simulink model "MSDRPrimaryLoop_LoadFollow"  (R2021b)
settings: Solver=VariableStepAuto  StartTime=0.0  StopTime=604900  MaxStep=1  MinStep=0.01  RelTol=1e-3
undefined symbols (not defined in the file): a_f, A_free_PHX, a_g, A_h_PHX, beta, beta_t, bubbleGeneratorArea, bubbleGeneratorDh, bubbleGeneratorElevation, bubbleGeneratorLength, bubbleGeneratorVolume, bubbleSaturationLevel, bubbleSeparatorArea, bubbleSeparatorDiameter, bubbleSeparatorDo, bubbleSeparatorLength, bubbleSeparatorSlope, bypassRatio, C0, coreFlowArea, coreFuelVolume, coreLowerPlenumArea, coreLowerPlenumHydraulicDiameter, coreLowerPlenumLength, coreLowerPlenumVolume, coreUpperPlenumArea, coreUpperPlenumHydraulicDiameter, coreUpperPlenumLength, coreUpperPlenumVolume, coreVolume, cpGraphite, dissolusionRatio, dMin, dScale, dsmConst, DXeG, Fiss_factor, fuelChannelHydrualicDiameter, fuelChannelLength, fuelDepositRatio, fuelFraction, fuelGraphiteArea, fuelGraphiteHeatTransferCoefficient, gamma0, gamma1, gamma2, generatorDsm, graphiteKDiff, graphiteUnitCellThickness, initialIodineConcentration, InitialXeMolarConcentration, InjectionRatio, injectionRatio, iodineDecayConstant, IodineDecayConstant, iodineYield, kGraphite, kScale, Lam, lam ... (+60)
libraries: fl_lib x268, nesl_utility x106, SimscapeFluids_lib x20, slpidlib x1
(part 4 of 12)

== system MSDRPrimaryLoop_LoadFollow/pipeReactorToPump/PLossFunc ==
  Constant : Constant  Value=Elevation*9.82
  PS-Simulink Converter : nesl_utility/PS-Simulink Converter  PhysicalDomain=network_engine_domain  SubClassName=ps_output  LeftPortType=input  RightPortType=output  PseudoPeriodic=off  Frequencies=[]  Unit=inherit  AffineConversion=off
      settings: SourceProductBaseCode=PW,SS
  PS-Simulink Converter1 : nesl_utility/PS-Simulink Converter  PhysicalDomain=network_engine_domain  SubClassName=ps_output  LeftPortType=input  RightPortType=output  PseudoPeriodic=off  Frequencies=[]  Unit=inherit  AffineConversion=off
      settings: SourceProductBaseCode=PW,SS
  Pressure & Temperature Sensor (TL) : fl_lib/Thermal Liquid/Sensors/Pressure & Temperature Sensor (TL)
      settings: SourceProductBaseCode=SS  InternalSimscapePortConfiguration="{\"Bottom\":[],\"Left\":[{\"id\":\"A\",\"label\":\"A\",\"type\":\"foundation.thermal_liquid.thermal_liquid\"}],\"Right\":[{\"id\":\"B\",\"label\":\"B\",\"type\":\"foundation.thermal_liquid.thermal_liquid\"},{\"id\":\"P\",\"label\":\"P\",\"type\":\"output\"},{\"id\":\"T\",\"label\":\"T\",\"type\":\"output\"}],\"Top\":[]}"
  Product : Product
  Subtract : Sum  Inputs=+-
  Thermodynamic Properties Sensor (TL) : fl_lib/Thermal Liquid/Sensors/Thermodynamic Properties Sensor (TL)
      settings: SourceProductBaseCode=SS  InternalSimscapePortConfiguration="{\"Bottom\":[],\"Left\":[{\"id\":\"A\",\"label\":\"A\",\"type\":\"foundation.thermal_liquid.thermal_liquid\"}],\"Right\":[{\"id\":\"U\",\"label\":\"u\",\"type\":\"output\"},{\"id\":\"RHO\",\"label\":\"rho\",\"type\":\"output\"},{\"id\":\"CP\",\"label\":\"cp\",\"type\":\"output\"}],\"Top\":[]}"
  Ref1 : PMIOPort  Side=Left
  Ref2 : PMIOPort  Port=2  Side=Right
  PLoss : Outport
  wires:
  PS-Simulink Converter1/1 -> Product/1
  PS-Simulink Converter/1 -> Subtract/1
  Product/1 -> Subtract/2
  Constant/1 -> Product/2
  Subtract/1 -> PLoss/1
  connections:
  Thermodynamic Properties Sensor (TL)/LConn1 -- Pressure & Temperature Sensor (TL)/RConn1 -- Ref2/RConn1
  PS-Simulink Converter/LConn1 -- Pressure & Temperature Sensor (TL)/RConn2
  Thermodynamic Properties Sensor (TL)/RConn2 -- PS-Simulink Converter1/LConn1
  Pressure & Temperature Sensor (TL)/LConn1 -- Ref1/RConn1

== system MSDRPrimaryLoop_LoadFollow/pipeReactorToPump/Subsystem ==
  note: Dh
  note: Dh
  note: Dh
  GasInRef : Inport
  2PModification : Subsystem  ReferencedSubsystem=TwoPhaseModification
      settings: PortSchema="{\"entries\":[{\"content\":{\"sides\":[{\"content\":{\"connectorIds\":[\"LConn1\"]},\"type\":\"ConnectorPlacement.EquallySpacedRectSide\",\"uuid\":\"7546b4b7-b669-49c8-8f27-f696391ea3ad\"},{\"content\":{\"connectorIds\":[\"RConn1\"],\"side\":\"RIGHT\"},\"type\":\"ConnectorPlacement.EquallySpacedRectSide\",\"uuid\":\"0e6176f2-177c-4327-bcfa-9a190fe9083f\"},{\"content\":{\"connectorIds\":[\"LConn2\"],\"side\":\"TOP\"},\"type\":\"ConnectorPlacement.EquallySpacedRectSide\",\"uuid\":\"16faf74c-4635-4009-a5b3-33dd03b625c6\"},{\"content\":{\"connectorIds\":[\"RConn2\",\"In1\"],\"side\":\"BOTTOM\"},\"type\":\"ConnectorPlacement.EquallySpacedRectSide\",\"uuid\":\"2081d73b-bb08-4ad9-b5c8-e48a4e9c4e20\"}]},\"type\":\"ConnectorPlacement.EquallySpacedConnector\",\"uuid\":\"243e4075-206b-4747-a8bc-b8f10d9a577f\"}],\"packageUris\":[\"http://schema.mathworks.com/mf0/Connector/R2020b\"],\"version\":\"1.0\"}"
  PS Abs : fl_lib/Physical Signals/Nonlinear Operators/PS Abs
      settings: SourceProductBaseCode=SS  InternalSimscapePortConfiguration="{\"Bottom\":[],\"Left\":[{\"id\":\"I\",\"label\":\"\",\"type\":\"input\"}],\"Right\":[{\"id\":\"O\",\"label\":\"\",\"type\":\"output\"}],\"Top\":[]}"
  Pipe (TL) : SimscapeFluids_lib/Thermal Liquid/Pipes & Fittings/Pipe (TL)  dynamic_compressibility=simscape.enum.onoff.on  inertia=simscape.enum.onoff.on  num_segments=1  pipe_length=Length m  area=Area m^2  Dh=0.1128 m  wall_spec=fluids.thermal_liquid.pipes_fittings.enum.wall_spec.rigid  Dh_rigid=Dh m  wall_compliance=1.2e-6 m/MPa  wall_time_constant=0.01 s  elevation_spec=foundation.enum.constant_variable.constant  elevation_gain=Elevation m  g=9.82 m/s^2  pressure_loss_spec=fluids.thermal_liquid.pipes_fittings.enum.PressureLossSpec.Haaland  length_add=1 m  roughness=15e-6 m  Re_friction_TLU=[400, 1000, 1500, 3000, 4000, 6000, 10000, 20000, 40000, 60000, 100000, 100000000]  friction_factor_TLU=[.264, .112, .071, .0417, .0387, .0268, .025, .0232, .0226, .022, .0214, .0214]  shape_factor=64  Re_lam=2000  Re_tur=4000  mdot_nominal=[.1, 1] kg/s  p_diff_nominal=[.001, .01] MPa  mdot_threshold=1e-6 kg/s  heat_transfer_spec=fluids.thermal_liquid.pipes_fittings.enum.HeatTransferSpec.Gnielinski  mdot_nominal_heat=[.1, 1] kg/s  T_in_nominal=[293.15, 293.15] K  T_out_nominal=[300, 300] K  p_in_nominal_heat=[.101325, .101325] MPa  T_wall_nominal=[303.15, 303.15] K  a_coeff=0.023  b_Re_power=0.8  c_Pr_power=0.4  Nu_lam=3.66  Re_Colburn_TLU=[100, 150, 1000]  Colburn_factor_TLU=[.019, .013, .002]  Re_Nu_TLU=[100, 150, 1000]  Pr_Nu_TLU=[1, 10]  Nu_TLU=[3.72, 4.21; 3.75, 4.44; 4.21, 7.15]  T0_vec=T0 K  p0_vec=P0 Pa  mdot0=0.1 kg/s
      settings: SourceProductBaseCode=SH  LogSimulationData=on
  Volumetric Flow Rate Sensor (TL) : fl_lib/Thermal Liquid/Sensors/Volumetric Flow Rate Sensor (TL)
      settings: SourceProductBaseCode=SS  InternalSimscapePortConfiguration="{\"Bottom\":[],\"Left\":[{\"id\":\"A\",\"label\":\"A\",\"type\":\"foundation.thermal_liquid.thermal_liquid\"}],\"Right\":[{\"id\":\"B\",\"label\":\"B\",\"type\":\"foundation.thermal_liquid.thermal_liquid\"},{\"id\":\"V\",\"label\":\"V\",\"type\":\"output\"}],\"Top\":[]}"
  Inlet : PMIOPort  Side=Left
  Outlet : PMIOPort  Port=2  Side=Right
  VolumeRate : PMIOPort  Port=3  Side=Right
  wires:
  GasInRef/1 -> 2PModification/1
  connections:
  Volumetric Flow Rate Sensor (TL)/RConn1 -- Pipe (TL)/LConn1
  2PModification/LConn2 -- Inlet/RConn1 -- Volumetric Flow Rate Sensor (TL)/LConn1
  Pipe (TL)/RConn1 -- 2PModification/RConn2 -- 2PModification/LConn1
  Volumetric Flow Rate Sensor (TL)/RConn2 -- PS Abs/LConn1
  PS Abs/RConn1 -- VolumeRate/RConn1
  2PModification/RConn1 -- Outlet/RConn1

== system MSDRPrimaryLoop_LoadFollow/pipeReactorToPump/XenonCalc ==
  XeIn : Inport  OutDataTypeStr=double  Unit=kg/s
  PLoss : Inport  Port=2
  GasRef : Inport  Port=3
  Absolute Reference (TL) : fl_lib/Thermal Liquid/Elements/Absolute Reference (TL)
      settings: SourceProductBaseCode=SS
  Demux : Demux  Outputs=2
  Gas : Subsystem
      settings: PortSchema="{\"entries\":[{\"content\":{\"sides\":[{\"content\":{\"connectorIds\":[\"In1\"]},\"type\":\"ConnectorPlacement.EquallySpacedRectSide\",\"uuid\":\"9457d014-8c8c-4ede-953a-dad1b8fcff2e\"},{\"content\":{\"connectorIds\":[\"Out1\"],\"side\":\"RIGHT\"},\"type\":\"ConnectorPlacement.EquallySpacedRectSide\",\"uuid\":\"6b13e550-1648-4662-a58b-f6f49b8dfc45\"},{\"content\":{\"connectorIds\":[\"Out2\",\"In2\"],\"side\":\"TOP\"},\"type\":\"ConnectorPlacement.EquallySpacedRectSide\",\"uuid\":\"73a4211d-b4c2-4f72-9c26-6ee46c1777bd\"},{\"content\":{\"connectorIds\":[\"In3\",\"In4\"],\"side\":\"BOTTOM\"},\"type\":\"ConnectorPlacement.EquallySpacedRectSide\",\"uuid\":\"ca62b0cd-46c8-418f-9a8b-9558726bf444\"}]},\"type\":\"ConnectorPlacement.EquallySpacedConnector\",\"uuid\":\"020f2da1-56fe-4a8a-8a2d-2f75d9123e14\"}],\"packageUris\":[\"http://schema.mathworks.com/mf0/Connector/R2020b\"],\"version\":\"1.0\"}"
  InterphaseTranfser : Subsystem
      settings: PortSchema="{\"entries\":[{\"content\":{\"sides\":[{\"content\":{\"connectorIds\":[\"In1\",\"In2\",\"In3\"]},\"type\":\"ConnectorPlacement.EquallySpacedRectSide\",\"uuid\":\"d6303689-138e-451a-a3c3-60d601b4795c\"},{\"content\":{\"connectorIds\":[\"In5\",\"Out1\"],\"side\":\"RIGHT\"},\"type\":\"ConnectorPlacement.EquallySpacedRectSide\",\"uuid\":\"e99266db-1ad9-4248-a3a9-dc80edd4cbf2\"},{\"content\":{\"connectorIds\":[\"LConn1\"],\"side\":\"TOP\"},\"type\":\"ConnectorPlacement.EquallySpacedRectSide\",\"uuid\":\"07679a3e-e535-452f-8d16-cac9376cf8bb\"},{\"content\":{\"connectorIds\":[\"In4\"],\"side\":\"BOTTOM\"},\"type\":\"ConnectorPlacement.EquallySpacedRectSide\",\"uuid\":\"cd334689-6a33-4cbf-8721-40055306f60f\"}]},\"type\":\"ConnectorPlacement.EquallySpacedConnector\",\"uuid\":\"2a8870ca-366d-4312-85a0-e0a2095078d0\"}],\"packageUris\":[\"http://schema.mathworks.com/mf0/Connector/R2020b\"],\"version\":\"1.0\"}"
  Mux : Mux  Inputs=2
  PS Abs : fl_lib/Physical Signals/Nonlinear Operators/PS Abs
      settings: SourceProductBaseCode=SS  InternalSimscapePortConfiguration="{\"Bottom\":[],\"Left\":[{\"id\":\"I\",\"label\":\"\",\"type\":\"input\"}],\"Right\":[{\"id\":\"O\",\"label\":\"\",\"type\":\"output\"}],\"Top\":[]}"
  PS-Simulink Converter : nesl_utility/PS-Simulink Converter  PhysicalDomain=network_engine_domain  SubClassName=ps_output  LeftPortType=input  RightPortType=output  PseudoPeriodic=off  Frequencies=[]  Unit=inherit  AffineConversion=off
      settings: SourceProductBaseCode=PW,SS
  PS-Simulink Converter1 : nesl_utility/PS-Simulink Converter  PhysicalDomain=network_engine_domain  SubClassName=ps_output  LeftPortType=input  RightPortType=output  PseudoPeriodic=off  Frequencies=[]  Unit=inherit  AffineConversion=off
      settings: SourceProductBaseCode=PW,SS
  Pressure & Temperature Sensor (TL) : fl_lib/Thermal Liquid/Sensors/Pressure & Temperature Sensor (TL)
      settings: SourceProductBaseCode=SS  InternalSimscapePortConfiguration="{\"Bottom\":[],\"Left\":[{\"id\":\"A\",\"label\":\"A\",\"type\":\"foundation.thermal_liquid.thermal_liquid\"}],\"Right\":[{\"id\":\"B\",\"label\":\"B\",\"type\":\"foundation.thermal_liquid.thermal_liquid\"},{\"id\":\"P\",\"label\":\"P\",\"type\":\"output\"},{\"id\":\"T\",\"label\":\"T\",\"type\":\"output\"}],\"Top\":[]}"
  Salt : Subsystem
      settings: PortSchema="{\"entries\":[{\"content\":{\"sides\":[{\"content\":{\"connectorIds\":[\"In1\",\"In2\",\"In3\"]},\"type\":\"ConnectorPlacement.EquallySpacedRectSide\",\"uuid\":\"9457d014-8c8c-4ede-953a-dad1b8fcff2e\"},{\"content\":{\"connectorIds\":[\"Out1\"],\"side\":\"RIGHT\"},\"type\":\"ConnectorPlacement.EquallySpacedRectSide\",\"uuid\":\"6b13e550-1648-4662-a58b-f6f49b8dfc45\"},{\"content\":{\"connectorIds\":[\"In4\",\"In5\"],\"side\":\"TOP\"},\"type\":\"ConnectorPlacement.EquallySpacedRectSide\",\"uuid\":\"73a4211d-b4c2-4f72-9c26-6ee46c1777bd\"},{\"content\":{\"connectorIds\":[\"Out2\",\"In6\"],\"side\":\"BOTTOM\"},\"type\":\"ConnectorPlacement.EquallySpacedRectSide\",\"uuid\":\"ca62b0cd-46c8-418f-9a8b-9558726bf444\"}]},\"type\":\"ConnectorPlacement.EquallySpacedConnector\",\"uuid\":\"020f2da1-56fe-4a8a-8a2d-2f75d9123e14\"}],\"packageUris\":[\"http://schema.mathworks.com/mf0/Connector/R2020b\"],\"version\":\"1.0\"}"
  Volumetric Flow Rate Sensor (TL) : fl_lib/Thermal Liquid/Sensors/Volumetric Flow Rate Sensor (TL)
      settings: SourceProductBaseCode=SS  InternalSimscapePortConfiguration="{\"Bottom\":[],\"Left\":[{\"id\":\"A\",\"label\":\"A\",\"type\":\"foundation.thermal_liquid.thermal_liquid\"}],\"Right\":[{\"id\":\"B\",\"label\":\"B\",\"type\":\"foundation.thermal_liquid.thermal_liquid\"},{\"id\":\"V\",\"label\":\"V\",\"type\":\"output\"}],\"Top\":[]}"
  Inlet : PMIOPort  Side=Left
  Outlet : PMIOPort  Port=2  Side=Right
  XeOut : Outport
  wires:
  XeIn/1 -> Demux/1
  PS-Simulink Converter/1 -> InterphaseTranfser/5(VolumeRate), Gas/4(VolumeRate), Salt/5(VolumeRate)
  GasRef/1 -> Gas/3(GasRef), InterphaseTranfser/2(GasRef), Salt/4(GasRef)
  Demux/1 -> Salt/1(XeLIn)
  [IodineSNDensity] -> Salt/2(IodineSNumberDensity)
  Demux/2 -> Gas/1(XeGIn)
  Salt/1(XeLOut) -> Mux/1
  Gas/1(XeGOut) -> Mux/2
  Mux/1 -> XeOut/1
  Salt/2(GxSalt) -> InterphaseTranfser/1(GxSalt)
  Gas/2(GxGas) -> InterphaseTranfser/3(GxGas)
  InterphaseTranfser/1(TranfserRate) -> Salt/6(Interphase), Gas/2(Interphase)
  PS-Simulink Converter1/1 -> Salt/3(T_f_ave)
  PLoss/1 -> InterphaseTranfser/4(PLoss)
  connections:
  Outlet/RConn1 -- Volumetric Flow Rate Sensor (TL)/RConn1 -- InterphaseTranfser/LConn1
  Volumetric Flow Rate Sensor (TL)/LConn1 -- Pressure & Temperature Sensor (TL)/LConn1 -- Inlet/RConn1
  Volumetric Flow Rate Sensor (TL)/RConn2 -- PS Abs/LConn1
  PS Abs/RConn1 -- PS-Simulink Converter/LConn1
  Pressure & Temperature Sensor (TL)/RConn1 -- Absolute Reference (TL)/LConn1
  Pressure & Temperature Sensor (TL)/RConn3 -- PS-Simulink Converter1/LConn1

== system MSDRPrimaryLoop_LoadFollow/Chemical Processing/Bubble Generator/GasCalc ==
  note: There is an issue over how we should implement the gas injection rate.
      | Using acutal physical model here could cause some instablity, as the separator efficiency also depends on the void fraction.
  GasIn : Inport
  Add : Sum  Inputs=++-
  Constant : Constant  Value=0
  Constant1 : Constant  Value=VoidFraction
  GasExpansion : Subsystem  ReferencedSubsystem=GasExpansion
      settings: PortSchema="{\"entries\":[{\"content\":{\"sides\":[{\"content\":{\"connectorIds\":[\"LConn1\",\"In1\"]},\"type\":\"ConnectorPlacement.EquallySpacedRectSide\",\"uuid\":\"50c89675-cb8a-4964-af62-cb2014507b1d\"},{\"content\":{\"connectorIds\":[\"RConn1\",\"Out1\"],\"side\":\"RIGHT\"},\"type\":\"ConnectorPlacement.EquallySpacedRectSide\",\"uuid\":\"6b3adc78-0be5-4682-9da0-6fd41ffc4e71\"},{\"content\":{\"connectorIds\":[],\"side\":\"TOP\"},\"type\":\"ConnectorPlacement.EquallySpacedRectSide\",\"uuid\":\"5158b46f-a496-48e4-90d6-6c6dcc9e237b\"}]},\"type\":\"ConnectorPlacement.EquallySpacedConnector\",\"uuid\":\"7ff0188e-dc19-44a0-a8cf-bde33949414f\"}],\"packageUris\":[\"http://schema.mathworks.com/mf0/Connector/R2020b\"],\"version\":\"1.0\"}"
  Integrator : Integrator
  Max : MinMax  Function=max  Inputs=2
  Minus : Sum  Inputs=+-
  PS-Simulink Converter : nesl_utility/PS-Simulink Converter  PhysicalDomain=network_engine_domain  SubClassName=ps_output  LeftPortType=input  RightPortType=output  PseudoPeriodic=off  Frequencies=[]  Unit=inherit  AffineConversion=off
      settings: SourceProductBaseCode=PW,SS
  Product : Product
  Product1 : Product
  Step : Step  Time=150  SampleTime=0
  VolumeToVoid : Gain  Gain=1/Volume
  Ref1 : PMIOPort  Side=Left
  VolumeRate : PMIOPort  Port=2  Side=Left
  Ref2 : PMIOPort  Port=3  Side=Left
  GasOut : Outport
  wires:
  VolumeToVoid/1 -> Add/3, GasExpansion/1
  Integrator/1 -> VolumeToVoid/1
  GasIn/1 -> Add/1, Minus/2
  Add/1 -> Product/1
  Product/1 -> Integrator/1
  PS-Simulink Converter/1 -> Product/2
  GasExpansion/1 -> GasOut/1
  Minus/1 -> Max/1
  Constant/1 -> Max/2
  Max/1 -> Add/2
  Constant1/1 -> Product1/1
  Step/1 -> Product1/2
  Product1/1 -> Minus/1
  connections:
  PS-Simulink Converter/LConn1 -- VolumeRate/RConn1
  GasExpansion/LConn1 -- Ref1/RConn1
  GasExpansion/RConn1 -- Ref2/RConn1

== system MSDRPrimaryLoop_LoadFollow/Chemical Processing/Bubble Generator/PLossFunc ==
  Constant : Constant  Value=bubbleGeneratorElevation*9.82
  PS-Simulink Converter : nesl_utility/PS-Simulink Converter  PhysicalDomain=network_engine_domain  SubClassName=ps_output  LeftPortType=input  RightPortType=output  PseudoPeriodic=off  Frequencies=[]  Unit=inherit  AffineConversion=off
      settings: SourceProductBaseCode=PW,SS
  PS-Simulink Converter1 : nesl_utility/PS-Simulink Converter  PhysicalDomain=network_engine_domain  SubClassName=ps_output  LeftPortType=input  RightPortType=output  PseudoPeriodic=off  Frequencies=[]  Unit=inherit  AffineConversion=off
      settings: SourceProductBaseCode=PW,SS
  Pressure & Temperature Sensor (TL) : fl_lib/Thermal Liquid/Sensors/Pressure & Temperature Sensor (TL)
      settings: SourceProductBaseCode=SS  InternalSimscapePortConfiguration="{\"Bottom\":[],\"Left\":[{\"id\":\"A\",\"label\":\"A\",\"type\":\"foundation.thermal_liquid.thermal_liquid\"}],\"Right\":[{\"id\":\"B\",\"label\":\"B\",\"type\":\"foundation.thermal_liquid.thermal_liquid\"},{\"id\":\"P\",\"label\":\"P\",\"type\":\"output\"},{\"id\":\"T\",\"label\":\"T\",\"type\":\"output\"}],\"Top\":[]}"
  Product : Product
  Subtract : Sum  Inputs=+-
  Thermodynamic Properties Sensor (TL) : fl_lib/Thermal Liquid/Sensors/Thermodynamic Properties Sensor (TL)
      settings: SourceProductBaseCode=SS  InternalSimscapePortConfiguration="{\"Bottom\":[],\"Left\":[{\"id\":\"A\",\"label\":\"A\",\"type\":\"foundation.thermal_liquid.thermal_liquid\"}],\"Right\":[{\"id\":\"U\",\"label\":\"u\",\"type\":\"output\"},{\"id\":\"RHO\",\"label\":\"rho\",\"type\":\"output\"},{\"id\":\"CP\",\"label\":\"cp\",\"type\":\"output\"}],\"Top\":[]}"
  Ref1 : PMIOPort  Side=Left
  Ref2 : PMIOPort  Port=2  Side=Right
  PLoss : Outport
  wires:
  PS-Simulink Converter1/1 -> Product/1
  PS-Simulink Converter/1 -> Subtract/1
  Product/1 -> Subtract/2
  Constant/1 -> Product/2
  Subtract/1 -> PLoss/1
  connections:
  Thermodynamic Properties Sensor (TL)/LConn1 -- Pressure & Temperature Sensor (TL)/RConn1 -- Ref2/RConn1
  PS-Simulink Converter/LConn1 -- Pressure & Temperature Sensor (TL)/RConn2
  Thermodynamic Properties Sensor (TL)/RConn2 -- PS-Simulink Converter1/LConn1
  Pressure & Temperature Sensor (TL)/LConn1 -- Ref1/RConn1

== system MSDRPrimaryLoop_LoadFollow/Chemical Processing/Bubble Generator/Subsystem ==
  note: Sudden Area change removed for good convergence. Probably not a big deal.
  note: Dh
  GasInRef : Inport
  2PModification : Subsystem  ReferencedSubsystem=TwoPhaseModification
      settings: PortSchema="{\"entries\":[{\"content\":{\"sides\":[{\"content\":{\"connectorIds\":[\"LConn1\"]},\"type\":\"ConnectorPlacement.EquallySpacedRectSide\",\"uuid\":\"7546b4b7-b669-49c8-8f27-f696391ea3ad\"},{\"content\":{\"connectorIds\":[\"RConn1\"],\"side\":\"RIGHT\"},\"type\":\"ConnectorPlacement.EquallySpacedRectSide\",\"uuid\":\"0e6176f2-177c-4327-bcfa-9a190fe9083f\"},{\"content\":{\"connectorIds\":[\"LConn2\"],\"side\":\"TOP\"},\"type\":\"ConnectorPlacement.EquallySpacedRectSide\",\"uuid\":\"16faf74c-4635-4009-a5b3-33dd03b625c6\"},{\"content\":{\"connectorIds\":[\"RConn2\",\"In1\"],\"side\":\"BOTTOM\"},\"type\":\"ConnectorPlacement.EquallySpacedRectSide\",\"uuid\":\"2081d73b-bb08-4ad9-b5c8-e48a4e9c4e20\"}]},\"type\":\"ConnectorPlacement.EquallySpacedConnector\",\"uuid\":\"243e4075-206b-4747-a8bc-b8f10d9a577f\"}],\"packageUris\":[\"http://schema.mathworks.com/mf0/Connector/R2020b\"],\"version\":\"1.0\"}"
  PS Abs : fl_lib/Physical Signals/Nonlinear Operators/PS Abs
      settings: SourceProductBaseCode=SS  InternalSimscapePortConfiguration="{\"Bottom\":[],\"Left\":[{\"id\":\"I\",\"label\":\"\",\"type\":\"input\"}],\"Right\":[{\"id\":\"O\",\"label\":\"\",\"type\":\"output\"}],\"Top\":[]}"
  Pipe (TL) : SimscapeFluids_lib/Thermal Liquid/Pipes & Fittings/Pipe (TL)  dynamic_compressibility=simscape.enum.onoff.on  inertia=simscape.enum.onoff.off  num_segments=1  pipe_length=Length m  area=Area m^2  Dh=Dh m  wall_spec=fluids.thermal_liquid.pipes_fittings.enum.wall_spec.rigid  Dh_rigid=Dh m  wall_compliance=1.2e-6 m/MPa  wall_time_constant=0.01 s  elevation_spec=foundation.enum.constant_variable.constant  elevation_gain=Elevation m  g=9.82 m/s^2  pressure_loss_spec=fluids.thermal_liquid.pipes_fittings.enum.PressureLossSpec.Haaland  length_add=1 m  roughness=15e-6 m  Re_friction_TLU=[400, 1000, 1500, 3000, 4000, 6000, 10000, 20000, 40000, 60000, 100000, 100000000]  friction_factor_TLU=[.264, .112, .071, .0417, .0387, .0268, .025, .0232, .0226, .022, .0214, .0214]  shape_factor=64  Re_lam=2000  Re_tur=4000  mdot_nominal=[.1, 1] kg/s  p_diff_nominal=[.001, .01] MPa  mdot_threshold=1e-6 kg/s  heat_transfer_spec=fluids.thermal_liquid.pipes_fittings.enum.HeatTransferSpec.Gnielinski  mdot_nominal_heat=[.1, 1] kg/s  T_in_nominal=[293.15, 293.15] K  T_out_nominal=[300, 300] K  p_in_nominal_heat=[.101325, .101325] MPa  T_wall_nominal=[303.15, 303.15] K  a_coeff=0.023  b_Re_power=0.8  c_Pr_power=0.4  Nu_lam=3.66  Re_Colburn_TLU=[100, 150, 1000]  Colburn_factor_TLU=[.019, .013, .002]  Re_Nu_TLU=[100, 150, 1000]  Pr_Nu_TLU=[1, 10]  Nu_TLU=[3.72, 4.21; 3.75, 4.44; 4.21, 7.15]  T0_vec=T0 K  p0_vec=P0 Pa  mdot0=0.1 kg/s
      settings: SourceProductBaseCode=SH  LogSimulationData=on
  Volumetric Flow Rate Sensor (TL) : fl_lib/Thermal Liquid/Sensors/Volumetric Flow Rate Sensor (TL)
      settings: SourceProductBaseCode=SS  InternalSimscapePortConfiguration="{\"Bottom\":[],\"Left\":[{\"id\":\"A\",\"label\":\"A\",\"type\":\"foundation.thermal_liquid.thermal_liquid\"}],\"Right\":[{\"id\":\"B\",\"label\":\"B\",\"type\":\"foundation.thermal_liquid.thermal_liquid\"},{\"id\":\"V\",\"label\":\"V\",\"type\":\"output\"}],\"Top\":[]}"
  Inlet : PMIOPort  Side=Left
  Outlet : PMIOPort  Port=2  Side=Right
  VolumeRate : PMIOPort  Port=3  Side=Right
  wires:
  GasInRef/1 -> 2PModification/1
  connections:
  Volumetric Flow Rate Sensor (TL)/RConn1 -- Pipe (TL)/LConn1
  Inlet/RConn1 -- 2PModification/LConn2 -- Volumetric Flow Rate Sensor (TL)/LConn1
  Volumetric Flow Rate Sensor (TL)/RConn2 -- PS Abs/LConn1
  PS Abs/RConn1 -- VolumeRate/RConn1
  2PModification/RConn1 -- Outlet/RConn1
  2PModification/LConn1 -- Pipe (TL)/RConn1 -- 2PModification/RConn2

== system MSDRPrimaryLoop_LoadFollow/Chemical Processing/Bubble Generator/XenonCalc ==
  XeIn : Inport  OutDataTypeStr=double  Unit=kg/s
  PLoss : Inport  Port=2
  GasRef : Inport  Port=3
  Absolute Reference (TL) : fl_lib/Thermal Liquid/Elements/Absolute Reference (TL)
      settings: SourceProductBaseCode=SS
  Demux : Demux  Outputs=2
  Gas : Subsystem
      settings: PortSchema="{\"entries\":[{\"content\":{\"sides\":[{\"content\":{\"connectorIds\":[\"In1\"]},\"type\":\"ConnectorPlacement.EquallySpacedRectSide\",\"uuid\":\"9457d014-8c8c-4ede-953a-dad1b8fcff2e\"},{\"content\":{\"connectorIds\":[\"Out1\"],\"side\":\"RIGHT\"},\"type\":\"ConnectorPlacement.EquallySpacedRectSide\",\"uuid\":\"6b13e550-1648-4662-a58b-f6f49b8dfc45\"},{\"content\":{\"connectorIds\":[\"Out2\",\"In2\"],\"side\":\"TOP\"},\"type\":\"ConnectorPlacement.EquallySpacedRectSide\",\"uuid\":\"73a4211d-b4c2-4f72-9c26-6ee46c1777bd\"},{\"content\":{\"connectorIds\":[\"In3\",\"In4\"],\"side\":\"BOTTOM\"},\"type\":\"ConnectorPlacement.EquallySpacedRectSide\",\"uuid\":\"ca62b0cd-46c8-418f-9a8b-9558726bf444\"}]},\"type\":\"ConnectorPlacement.EquallySpacedConnector\",\"uuid\":\"020f2da1-56fe-4a8a-8a2d-2f75d9123e14\"}],\"packageUris\":[\"http://schema.mathworks.com/mf0/Connector/R2020b\"],\"version\":\"1.0\"}"
  InterphaseTranfser : Subsystem
      settings: PortSchema="{\"entries\":[{\"content\":{\"sides\":[{\"content\":{\"connectorIds\":[\"In1\",\"In2\",\"In3\"]},\"type\":\"ConnectorPlacement.EquallySpacedRectSide\",\"uuid\":\"d6303689-138e-451a-a3c3-60d601b4795c\"},{\"content\":{\"connectorIds\":[\"In5\",\"Out1\"],\"side\":\"RIGHT\"},\"type\":\"ConnectorPlacement.EquallySpacedRectSide\",\"uuid\":\"e99266db-1ad9-4248-a3a9-dc80edd4cbf2\"},{\"content\":{\"connectorIds\":[\"LConn1\"],\"side\":\"TOP\"},\"type\":\"ConnectorPlacement.EquallySpacedRectSide\",\"uuid\":\"07679a3e-e535-452f-8d16-cac9376cf8bb\"},{\"content\":{\"connectorIds\":[\"In4\"],\"side\":\"BOTTOM\"},\"type\":\"ConnectorPlacement.EquallySpacedRectSide\",\"uuid\":\"cd334689-6a33-4cbf-8721-40055306f60f\"}]},\"type\":\"ConnectorPlacement.EquallySpacedConnector\",\"uuid\":\"2a8870ca-366d-4312-85a0-e0a2095078d0\"}],\"packageUris\":[\"http://schema.mathworks.com/mf0/Connector/R2020b\"],\"version\":\"1.0\"}"
  Mux : Mux  Inputs=2
  PS Abs : fl_lib/Physical Signals/Nonlinear Operators/PS Abs
      settings: SourceProductBaseCode=SS  InternalSimscapePortConfiguration="{\"Bottom\":[],\"Left\":[{\"id\":\"I\",\"label\":\"\",\"type\":\"input\"}],\"Right\":[{\"id\":\"O\",\"label\":\"\",\"type\":\"output\"}],\"Top\":[]}"
  PS-Simulink Converter : nesl_utility/PS-Simulink Converter  PhysicalDomain=network_engine_domain  SubClassName=ps_output  LeftPortType=input  RightPortType=output  PseudoPeriodic=off  Frequencies=[]  Unit=inherit  AffineConversion=off
      settings: SourceProductBaseCode=PW,SS
  PS-Simulink Converter1 : nesl_utility/PS-Simulink Converter  PhysicalDomain=network_engine_domain  SubClassName=ps_output  LeftPortType=input  RightPortType=output  PseudoPeriodic=off  Frequencies=[]  Unit=inherit  AffineConversion=off
      settings: SourceProductBaseCode=PW,SS
  Pressure & Temperature Sensor (TL) : fl_lib/Thermal Liquid/Sensors/Pressure & Temperature Sensor (TL)
      settings: SourceProductBaseCode=SS  InternalSimscapePortConfiguration="{\"Bottom\":[],\"Left\":[{\"id\":\"A\",\"label\":\"A\",\"type\":\"foundation.thermal_liquid.thermal_liquid\"}],\"Right\":[{\"id\":\"B\",\"label\":\"B\",\"type\":\"foundation.thermal_liquid.thermal_liquid\"},{\"id\":\"P\",\"label\":\"P\",\"type\":\"output\"},{\"id\":\"T\",\"label\":\"T\",\"type\":\"output\"}],\"Top\":[]}"
  Salt : Subsystem
      settings: PortSchema="{\"entries\":[{\"content\":{\"sides\":[{\"content\":{\"connectorIds\":[\"In1\",\"In2\",\"In3\"]},\"type\":\"ConnectorPlacement.EquallySpacedRectSide\",\"uuid\":\"9457d014-8c8c-4ede-953a-dad1b8fcff2e\"},{\"content\":{\"connectorIds\":[\"Out1\"],\"side\":\"RIGHT\"},\"type\":\"ConnectorPlacement.EquallySpacedRectSide\",\"uuid\":\"6b13e550-1648-4662-a58b-f6f49b8dfc45\"},{\"content\":{\"connectorIds\":[\"In4\",\"In5\"],\"side\":\"TOP\"},\"type\":\"ConnectorPlacement.EquallySpacedRectSide\",\"uuid\":\"73a4211d-b4c2-4f72-9c26-6ee46c1777bd\"},{\"content\":{\"connectorIds\":[\"Out2\",\"In6\"],\"side\":\"BOTTOM\"},\"type\":\"ConnectorPlacement.EquallySpacedRectSide\",\"uuid\":\"ca62b0cd-46c8-418f-9a8b-9558726bf444\"}]},\"type\":\"ConnectorPlacement.EquallySpacedConnector\",\"uuid\":\"020f2da1-56fe-4a8a-8a2d-2f75d9123e14\"}],\"packageUris\":[\"http://schema.mathworks.com/mf0/Connector/R2020b\"],\"version\":\"1.0\"}"
  Volumetric Flow Rate Sensor (TL) : fl_lib/Thermal Liquid/Sensors/Volumetric Flow Rate Sensor (TL)
      settings: SourceProductBaseCode=SS  InternalSimscapePortConfiguration="{\"Bottom\":[],\"Left\":[{\"id\":\"A\",\"label\":\"A\",\"type\":\"foundation.thermal_liquid.thermal_liquid\"}],\"Right\":[{\"id\":\"B\",\"label\":\"B\",\"type\":\"foundation.thermal_liquid.thermal_liquid\"},{\"id\":\"V\",\"label\":\"V\",\"type\":\"output\"}],\"Top\":[]}"
  Inlet : PMIOPort  Side=Left
  Outlet : PMIOPort  Port=2  Side=Right
  XeOut : Outport
  wires:
  XeIn/1 -> Demux/1
  PS-Simulink Converter/1 -> InterphaseTranfser/5(VolumeRate), Gas/4(VolumeRate), Salt/5(VolumeRate)
  GasRef/1 -> Gas/3(GasRef), InterphaseTranfser/2(GasRef), Salt/4(GasRef)
  Demux/1 -> Salt/1(XeLIn)
  [IodineSNDensity] -> Salt/2(IodineSNumberDensity)
  Demux/2 -> Gas/1(XeGIn)
  Salt/1(XeLOut) -> Mux/1
  Gas/1(XeGOut) -> Mux/2
  Mux/1 -> XeOut/1
  Salt/2(GxSalt) -> InterphaseTranfser/1(GxSalt)
  Gas/2(GxGas) -> InterphaseTranfser/3(GxGas)
  InterphaseTranfser/1(TranfserRate) -> Gas/2(Interphase), Salt/6(Interphase)
  PS-Simulink Converter1/1 -> Salt/3(T_f_ave)
  PLoss/1 -> InterphaseTranfser/4(PLoss)
  connections:
  Outlet/RConn1 -- Volumetric Flow Rate Sensor (TL)/RConn1 -- InterphaseTranfser/LConn1
  Volumetric Flow Rate Sensor (TL)/LConn1 -- Pressure & Temperature Sensor (TL)/LConn1 -- Inlet/RConn1
  Volumetric Flow Rate Sensor (TL)/RConn2 -- PS Abs/LConn1
  PS Abs/RConn1 -- PS-Simulink Converter/LConn1
  Pressure & Temperature Sensor (TL)/RConn1 -- Absolute Reference (TL)/LConn1
  Pressure & Temperature Sensor (TL)/RConn3 -- PS-Simulink Converter1/LConn1

== system MSDRPrimaryLoop_LoadFollow/Chemical Processing/Bubble Separator/Subsystem ==
  GasIn : Inport
  volRate : Inport  Port=2
  Constant : Constant
  Constitutive : Subsystem
      settings: PortSchema="{\"entries\":[{\"content\":{\"sides\":[{\"content\":{\"connectorIds\":[\"LConn1\",\"In1\"]},\"type\":\"ConnectorPlacement.EquallySpacedRectSide\",\"uuid\":\"b30af6c3-7c55-4661-bc76-939f1c8a4177\"},{\"content\":{\"connectorIds\":[\"Out1\",\"Out2\",\"Out3\",\"Out4\",\"Out5\",\"Out6\",\"Out7\",\"Out8\",\"Out9\",\"Out10\",\"Out11\"],\"side\":\"RIGHT\"},\"type\":\"ConnectorPlacement.EquallySpacedRectSide\",\"uuid\":\"0b137634-5e01-4bd6-8381-72b0699f5835\"},{\"content\":{\"connectorIds\":[],\"side\":\"TOP\"},\"type\":\"ConnectorPlacement.EquallySpacedRectSide\",\"uuid\":\"06046061-3240-493e-a0a3-282c9541adae\"}]},\"type\":\"ConnectorPlacement.EquallySpacedConnector\",\"uuid\":\"b0591291-fd4b-4355-beaa-e569a19c4b12\"}],\"packageUris\":[\"http://schema.mathworks.com/mf0/Connector/R2020b\"],\"version\":\"1.0\"}"
  MATLAB Function : MATLAB Function  TreatAsAtomicUnit=on
  Product : Product
  Subsystem : Subsystem  ReferencedSubsystem=GasToAlpha
  Subtract : Sum  Inputs=+-
  RefIn : PMIOPort  Side=Right
  GasOut : Outport
  SepEff : Outport  Port=2
  wires:
  GasIn/1 -> Product/1, Subsystem/1
  volRate/1 -> Constitutive/1(VolumeRate)
  Constitutive/1(rho) -> MATLAB Function/2(rho)
  Constitutive/2(ul) -> MATLAB Function/3(jl)
  Subsystem/1 -> MATLAB Function/1(alpha)
  Constitutive/11(dsm) -> MATLAB Function/12(dsm)
  Constitutive/3(dP) -> MATLAB Function/4(dP)
  Constitutive/4(Do) -> MATLAB Function/5(Do)
  Constitutive/5(Lsp) -> MATLAB Function/6(Lsp)
  Constitutive/6(D) -> MATLAB Function/7(D)
  Constitutive/7(Slope) -> MATLAB Function/8(k)
  Constitutive/8(Re) -> MATLAB Function/9(Re)
  Constitutive/9(sigma) -> MATLAB Function/10(sigma)
  Constitutive/10(mu) -> MATLAB Function/11(mu)
  Constant/1 -> Subtract/1
  MATLAB Function/1(separatorEfficiency) -> SepEff/1, Subtract/2
  Subtract/1 -> Product/2
  Product/1 -> GasOut/1
  connections:
  RefIn/RConn1 -- Constitutive/LConn1

== system MSDRPrimaryLoop_LoadFollow/Chemical Processing/ElevationPipe/GasCalc ==
  GasIn : Inport
  Add : Sum  Inputs=+-
  GasExpansion : Subsystem  ReferencedSubsystem=GasExpansion
      settings: PortSchema="{\"entries\":[{\"content\":{\"sides\":[{\"content\":{\"connectorIds\":[\"LConn1\",\"In1\"]},\"type\":\"ConnectorPlacement.EquallySpacedRectSide\",\"uuid\":\"50c89675-cb8a-4964-af62-cb2014507b1d\"},{\"content\":{\"connectorIds\":[\"RConn1\",\"Out1\"],\"side\":\"RIGHT\"},\"type\":\"ConnectorPlacement.EquallySpacedRectSide\",\"uuid\":\"6b3adc78-0be5-4682-9da0-6fd41ffc4e71\"},{\"content\":{\"connectorIds\":[],\"side\":\"TOP\"},\"type\":\"ConnectorPlacement.EquallySpacedRectSide\",\"uuid\":\"5158b46f-a496-48e4-90d6-6c6dcc9e237b\"}]},\"type\":\"ConnectorPlacement.EquallySpacedConnector\",\"uuid\":\"7ff0188e-dc19-44a0-a8cf-bde33949414f\"}],\"packageUris\":[\"http://schema.mathworks.com/mf0/Connector/R2020b\"],\"version\":\"1.0\"}"
  Integrator : Integrator
  PS-Simulink Converter : nesl_utility/PS-Simulink Converter  PhysicalDomain=network_engine_domain  SubClassName=ps_output  LeftPortType=input  RightPortType=output  PseudoPeriodic=off  Frequencies=[]  Unit=inherit  AffineConversion=off
      settings: SourceProductBaseCode=PW,SS
  Product : Product
  VolumeToVoid : Gain  Gain=1/Volume
  Ref1 : PMIOPort  Side=Left
  VolumeRate : PMIOPort  Port=2  Side=Left
  Ref2 : PMIOPort  Port=3  Side=Left
  GasOut : Outport
  wires:
  VolumeToVoid/1 -> GasExpansion/1, Add/2
  Integrator/1 -> VolumeToVoid/1
  GasIn/1 -> Add/1
  Add/1 -> Product/1
  Product/1 -> Integrator/1
  PS-Simulink Converter/1 -> Product/2
  GasExpansion/1 -> GasOut/1
  connections:
  PS-Simulink Converter/LConn1 -- VolumeRate/RConn1
  GasExpansion/LConn1 -- Ref1/RConn1
  GasExpansion/RConn1 -- Ref2/RConn1

== system MSDRPrimaryLoop_LoadFollow/Chemical Processing/ElevationPipe/PLossFunc ==
  Constant : Constant  Value=Elevation*9.82
  PS-Simulink Converter : nesl_utility/PS-Simulink Converter  PhysicalDomain=network_engine_domain  SubClassName=ps_output  LeftPortType=input  RightPortType=output  PseudoPeriodic=off  Frequencies=[]  Unit=inherit  AffineConversion=off
      settings: SourceProductBaseCode=PW,SS
  PS-Simulink Converter1 : nesl_utility/PS-Simulink Converter  PhysicalDomain=network_engine_domain  SubClassName=ps_output  LeftPortType=input  RightPortType=output  PseudoPeriodic=off  Frequencies=[]  Unit=inherit  AffineConversion=off
      settings: SourceProductBaseCode=PW,SS
  Pressure & Temperature Sensor (TL) : fl_lib/Thermal Liquid/Sensors/Pressure & Temperature Sensor (TL)
      settings: SourceProductBaseCode=SS  InternalSimscapePortConfiguration="{\"Bottom\":[],\"Left\":[{\"id\":\"A\",\"label\":\"A\",\"type\":\"foundation.thermal_liquid.thermal_liquid\"}],\"Right\":[{\"id\":\"B\",\"label\":\"B\",\"type\":\"foundation.thermal_liquid.thermal_liquid\"},{\"id\":\"P\",\"label\":\"P\",\"type\":\"output\"},{\"id\":\"T\",\"label\":\"T\",\"type\":\"output\"}],\"Top\":[]}"
  Product : Product
  Subtract : Sum  Inputs=+-
  Thermodynamic Properties Sensor (TL) : fl_lib/Thermal Liquid/Sensors/Thermodynamic Properties Sensor (TL)
      settings: SourceProductBaseCode=SS  InternalSimscapePortConfiguration="{\"Bottom\":[],\"Left\":[{\"id\":\"A\",\"label\":\"A\",\"type\":\"foundation.thermal_liquid.thermal_liquid\"}],\"Right\":[{\"id\":\"U\",\"label\":\"u\",\"type\":\"output\"},{\"id\":\"RHO\",\"label\":\"rho\",\"type\":\"output\"},{\"id\":\"CP\",\"label\":\"cp\",\"type\":\"output\"}],\"Top\":[]}"
  Ref1 : PMIOPort  Side=Left
  Ref2 : PMIOPort  Port=2  Side=Right
  PLoss : Outport
  wires:
  PS-Simulink Converter1/1 -> Product/1
  PS-Simulink Converter/1 -> Subtract/1
  Product/1 -> Subtract/2
  Constant/1 -> Product/2
  Subtract/1 -> PLoss/1
  connections:
  Thermodynamic Properties Sensor (TL)/LConn1 -- Pressure & Temperature Sensor (TL)/RConn1 -- Ref2/RConn1
  PS-Simulink Converter/LConn1 -- Pressure & Temperature Sensor (TL)/RConn2
  Thermodynamic Properties Sensor (TL)/RConn2 -- PS-Simulink Converter1/LConn1
  Pressure & Temperature Sensor (TL)/LConn1 -- Ref1/RConn1

== system MSDRPrimaryLoop_LoadFollow/Chemical Processing/ElevationPipe/Subsystem ==
  note: Dh
  note: Dh
  note: Dh
  GasInRef : Inport
  2PModification : Subsystem  ReferencedSubsystem=TwoPhaseModification
      settings: PortSchema="{\"entries\":[{\"content\":{\"sides\":[{\"content\":{\"connectorIds\":[\"LConn1\"]},\"type\":\"ConnectorPlacement.EquallySpacedRectSide\",\"uuid\":\"7546b4b7-b669-49c8-8f27-f696391ea3ad\"},{\"content\":{\"connectorIds\":[\"RConn1\"],\"side\":\"RIGHT\"},\"type\":\"ConnectorPlacement.EquallySpacedRectSide\",\"uuid\":\"0e6176f2-177c-4327-bcfa-9a190fe9083f\"},{\"content\":{\"connectorIds\":[\"LConn2\"],\"side\":\"TOP\"},\"type\":\"ConnectorPlacement.EquallySpacedRectSide\",\"uuid\":\"16faf74c-4635-4009-a5b3-33dd03b625c6\"},{\"content\":{\"connectorIds\":[\"RConn2\",\"In1\"],\"side\":\"BOTTOM\"},\"type\":\"ConnectorPlacement.EquallySpacedRectSide\",\"uuid\":\"2081d73b-bb08-4ad9-b5c8-e48a4e9c4e20\"}]},\"type\":\"ConnectorPlacement.EquallySpacedConnector\",\"uuid\":\"243e4075-206b-4747-a8bc-b8f10d9a577f\"}],\"packageUris\":[\"http://schema.mathworks.com/mf0/Connector/R2020b\"],\"version\":\"1.0\"}"
  PS Abs : fl_lib/Physical Signals/Nonlinear Operators/PS Abs
      settings: SourceProductBaseCode=SS  InternalSimscapePortConfiguration="{\"Bottom\":[],\"Left\":[{\"id\":\"I\",\"label\":\"\",\"type\":\"input\"}],\"Right\":[{\"id\":\"O\",\"label\":\"\",\"type\":\"output\"}],\"Top\":[]}"
  Pipe (TL) : SimscapeFluids_lib/Thermal Liquid/Pipes & Fittings/Pipe (TL)  dynamic_compressibility=simscape.enum.onoff.on  inertia=simscape.enum.onoff.off  num_segments=1  pipe_length=Length m  area=Area m^2  Dh=0.1128 m  wall_spec=fluids.thermal_liquid.pipes_fittings.enum.wall_spec.rigid  Dh_rigid=Dh m  wall_compliance=1.2e-6 m/MPa  wall_time_constant=0.01 s  elevation_spec=foundation.enum.constant_variable.constant  elevation_gain=Elevation m  g=9.82 m/s^2  pressure_loss_spec=fluids.thermal_liquid.pipes_fittings.enum.PressureLossSpec.Haaland  length_add=1 m  roughness=15e-6 m  Re_friction_TLU=[400, 1000, 1500, 3000, 4000, 6000, 10000, 20000, 40000, 60000, 100000, 100000000]  friction_factor_TLU=[.264, .112, .071, .0417, .0387, .0268, .025, .0232, .0226, .022, .0214, .0214]  shape_factor=64  Re_lam=2000  Re_tur=4000  mdot_nominal=[.1, 1] kg/s  p_diff_nominal=[.001, .01] MPa  mdot_threshold=1e-6 kg/s  heat_transfer_spec=fluids.thermal_liquid.pipes_fittings.enum.HeatTransferSpec.Gnielinski  mdot_nominal_heat=[.1, 1] kg/s  T_in_nominal=[293.15, 293.15] K  T_out_nominal=[300, 300] K  p_in_nominal_heat=[.101325, .101325] MPa  T_wall_nominal=[303.15, 303.15] K  a_coeff=0.023  b_Re_power=0.8  c_Pr_power=0.4  Nu_lam=3.66  Re_Colburn_TLU=[100, 150, 1000]  Colburn_factor_TLU=[.019, .013, .002]  Re_Nu_TLU=[100, 150, 1000]  Pr_Nu_TLU=[1, 10]  Nu_TLU=[3.72, 4.21; 3.75, 4.44; 4.21, 7.15]  T0_vec=T0 K  p0_vec=P0 Pa  mdot0=0.1 kg/s
      settings: SourceProductBaseCode=SH  LogSimulationData=on
  Volumetric Flow Rate Sensor (TL) : fl_lib/Thermal Liquid/Sensors/Volumetric Flow Rate Sensor (TL)
      settings: SourceProductBaseCode=SS  InternalSimscapePortConfiguration="{\"Bottom\":[],\"Left\":[{\"id\":\"A\",\"label\":\"A\",\"type\":\"foundation.thermal_liquid.thermal_liquid\"}],\"Right\":[{\"id\":\"B\",\"label\":\"B\",\"type\":\"foundation.thermal_liquid.thermal_liquid\"},{\"id\":\"V\",\"label\":\"V\",\"type\":\"output\"}],\"Top\":[]}"
  Inlet : PMIOPort  Side=Left
  Outlet : PMIOPort  Port=2  Side=Right
  VolumeRate : PMIOPort  Port=3  Side=Right
  wires:
  GasInRef/1 -> 2PModification/1
  connections:
  Volumetric Flow Rate Sensor (TL)/RConn1 -- Pipe (TL)/LConn1
  Inlet/RConn1 -- 2PModification/LConn2 -- Volumetric Flow Rate Sensor (TL)/LConn1
  Pipe (TL)/RConn1 -- 2PModification/LConn1 -- 2PModification/RConn2
  Volumetric Flow Rate Sensor (TL)/RConn2 -- PS Abs/LConn1
  PS Abs/RConn1 -- VolumeRate/RConn1
  2PModification/RConn1 -- Outlet/RConn1

== system MSDRPrimaryLoop_LoadFollow/Chemical Processing/ElevationPipe/XenonCalc ==
  XeIn : Inport  OutDataTypeStr=double  Unit=kg/s
  PLoss : Inport  Port=2
  GasRef : Inport  Port=3
  Absolute Reference (TL) : fl_lib/Thermal Liquid/Elements/Absolute Reference (TL)
      settings: SourceProductBaseCode=SS
  Demux : Demux  Outputs=2
  Gas : Subsystem
      settings: PortSchema="{\"entries\":[{\"content\":{\"sides\":[{\"content\":{\"connectorIds\":[\"In1\"]},\"type\":\"ConnectorPlacement.EquallySpacedRectSide\",\"uuid\":\"9457d014-8c8c-4ede-953a-dad1b8fcff2e\"},{\"content\":{\"connectorIds\":[\"Out1\"],\"side\":\"RIGHT\"},\"type\":\"ConnectorPlacement.EquallySpacedRectSide\",\"uuid\":\"6b13e550-1648-4662-a58b-f6f49b8dfc45\"},{\"content\":{\"connectorIds\":[\"Out2\",\"In2\"],\"side\":\"TOP\"},\"type\":\"ConnectorPlacement.EquallySpacedRectSide\",\"uuid\":\"73a4211d-b4c2-4f72-9c26-6ee46c1777bd\"},{\"content\":{\"connectorIds\":[\"In3\",\"In4\"],\"side\":\"BOTTOM\"},\"type\":\"ConnectorPlacement.EquallySpacedRectSide\",\"uuid\":\"ca62b0cd-46c8-418f-9a8b-9558726bf444\"}]},\"type\":\"ConnectorPlacement.EquallySpacedConnector\",\"uuid\":\"020f2da1-56fe-4a8a-8a2d-2f75d9123e14\"}],\"packageUris\":[\"http://schema.mathworks.com/mf0/Connector/R2020b\"],\"version\":\"1.0\"}"
  InterphaseTranfser1 : Subsystem
      settings: PortSchema="{\"entries\":[{\"content\":{\"sides\":[{\"content\":{\"connectorIds\":[\"In1\",\"In2\",\"In3\"]},\"type\":\"ConnectorPlacement.EquallySpacedRectSide\",\"uuid\":\"d6303689-138e-451a-a3c3-60d601b4795c\"},{\"content\":{\"connectorIds\":[\"In5\",\"Out1\"],\"side\":\"RIGHT\"},\"type\":\"ConnectorPlacement.EquallySpacedRectSide\",\"uuid\":\"e99266db-1ad9-4248-a3a9-dc80edd4cbf2\"},{\"content\":{\"connectorIds\":[\"LConn1\"],\"side\":\"TOP\"},\"type\":\"ConnectorPlacement.EquallySpacedRectSide\",\"uuid\":\"07679a3e-e535-452f-8d16-cac9376cf8bb\"},{\"content\":{\"connectorIds\":[\"In4\"],\"side\":\"BOTTOM\"},\"type\":\"ConnectorPlacement.EquallySpacedRectSide\",\"uuid\":\"cd334689-6a33-4cbf-8721-40055306f60f\"}]},\"type\":\"ConnectorPlacement.EquallySpacedConnector\",\"uuid\":\"2a8870ca-366d-4312-85a0-e0a2095078d0\"}],\"packageUris\":[\"http://schema.mathworks.com/mf0/Connector/R2020b\"],\"version\":\"1.0\"}"
  Mux : Mux  Inputs=2
  PS Abs : fl_lib/Physical Signals/Nonlinear Operators/PS Abs
      settings: SourceProductBaseCode=SS  InternalSimscapePortConfiguration="{\"Bottom\":[],\"Left\":[{\"id\":\"I\",\"label\":\"\",\"type\":\"input\"}],\"Right\":[{\"id\":\"O\",\"label\":\"\",\"type\":\"output\"}],\"Top\":[]}"
  PS-Simulink Converter : nesl_utility/PS-Simulink Converter  PhysicalDomain=network_engine_domain  SubClassName=ps_output  LeftPortType=input  RightPortType=output  PseudoPeriodic=off  Frequencies=[]  Unit=inherit  AffineConversion=off
      settings: SourceProductBaseCode=PW,SS
  PS-Simulink Converter1 : nesl_utility/PS-Simulink Converter  PhysicalDomain=network_engine_domain  SubClassName=ps_output  LeftPortType=input  RightPortType=output  PseudoPeriodic=off  Frequencies=[]  Unit=inherit  AffineConversion=off
      settings: SourceProductBaseCode=PW,SS
  Pressure & Temperature Sensor (TL) : fl_lib/Thermal Liquid/Sensors/Pressure & Temperature Sensor (TL)
      settings: SourceProductBaseCode=SS  InternalSimscapePortConfiguration="{\"Bottom\":[],\"Left\":[{\"id\":\"A\",\"label\":\"A\",\"type\":\"foundation.thermal_liquid.thermal_liquid\"}],\"Right\":[{\"id\":\"B\",\"label\":\"B\",\"type\":\"foundation.thermal_liquid.thermal_liquid\"},{\"id\":\"P\",\"label\":\"P\",\"type\":\"output\"},{\"id\":\"T\",\"label\":\"T\",\"type\":\"output\"}],\"Top\":[]}"
  Salt : Subsystem
      settings: PortSchema="{\"entries\":[{\"content\":{\"sides\":[{\"content\":{\"connectorIds\":[\"In1\",\"In2\",\"In3\"]},\"type\":\"ConnectorPlacement.EquallySpacedRectSide\",\"uuid\":\"9457d014-8c8c-4ede-953a-dad1b8fcff2e\"},{\"content\":{\"connectorIds\":[\"Out1\"],\"side\":\"RIGHT\"},\"type\":\"ConnectorPlacement.EquallySpacedRectSide\",\"uuid\":\"6b13e550-1648-4662-a58b-f6f49b8dfc45\"},{\"content\":{\"connectorIds\":[\"In4\",\"In5\"],\"side\":\"TOP\"},\"type\":\"ConnectorPlacement.EquallySpacedRectSide\",\"uuid\":\"73a4211d-b4c2-4f72-9c26-6ee46c1777bd\"},{\"content\":{\"connectorIds\":[\"Out2\",\"In6\"],\"side\":\"BOTTOM\"},\"type\":\"ConnectorPlacement.EquallySpacedRectSide\",\"uuid\":\"ca62b0cd-46c8-418f-9a8b-9558726bf444\"}]},\"type\":\"ConnectorPlacement.EquallySpacedConnector\",\"uuid\":\"020f2da1-56fe-4a8a-8a2d-2f75d9123e14\"}],\"packageUris\":[\"http://schema.mathworks.com/mf0/Connector/R2020b\"],\"version\":\"1.0\"}"
  Volumetric Flow Rate Sensor (TL) : fl_lib/Thermal Liquid/Sensors/Volumetric Flow Rate Sensor (TL)
      settings: SourceProductBaseCode=SS  InternalSimscapePortConfiguration="{\"Bottom\":[],\"Left\":[{\"id\":\"A\",\"label\":\"A\",\"type\":\"foundation.thermal_liquid.thermal_liquid\"}],\"Right\":[{\"id\":\"B\",\"label\":\"B\",\"type\":\"foundation.thermal_liquid.thermal_liquid\"},{\"id\":\"V\",\"label\":\"V\",\"type\":\"output\"}],\"Top\":[]}"
  Inlet : PMIOPort  Side=Left
  Outlet : PMIOPort  Port=2  Side=Right
  XeOut : Outport
  wires:
  XeIn/1 -> Demux/1
  PS-Simulink Converter/1 -> InterphaseTranfser1/5(VolumeRate), Gas/4(VolumeRate), Salt/5(VolumeRate)
  GasRef/1 -> InterphaseTranfser1/2(GasRef), Gas/3(GasRef), Salt/4(GasRef)
  Demux/1 -> Salt/1(XeLIn)
  [IodineSNDensity] -> Salt/2(IodineSNumberDensity)
  Demux/2 -> Gas/1(XeGIn)
  Salt/1(XeLOut) -> Mux/1
  Gas/1(XeGOut) -> Mux/2
  Mux/1 -> XeOut/1
  Salt/2(GxSalt) -> InterphaseTranfser1/1(GxSalt)
  Gas/2(GxGas) -> InterphaseTranfser1/3(GxGas)
  InterphaseTranfser1/1(TranfserRate) -> Salt/6(Interphase), Gas/2(Interphase)
  PS-Simulink Converter1/1 -> Salt/3(T_f_ave)
  PLoss/1 -> InterphaseTranfser1/4(PLoss)
  connections:
  Outlet/RConn1 -- InterphaseTranfser1/LConn1 -- Volumetric Flow Rate Sensor (TL)/RConn1
  Volumetric Flow Rate Sensor (TL)/LConn1 -- Pressure & Temperature Sensor (TL)/LConn1 -- Inlet/RConn1
  Volumetric Flow Rate Sensor (TL)/RConn2 -- PS Abs/LConn1
  PS Abs/RConn1 -- PS-Simulink Converter/LConn1
  Pressure & Temperature Sensor (TL)/RConn1 -- Absolute Reference (TL)/LConn1
  Pressure & Temperature Sensor (TL)/RConn3 -- PS-Simulink Converter1/LConn1

== system MSDRPrimaryLoop_LoadFollow/Chemical Processing/PipeLine/GasCalc ==
  GasIn : Inport
  Add : Sum  Inputs=+-
  GasExpansion : Subsystem  ReferencedSubsystem=GasExpansion
      settings: PortSchema="{\"entries\":[{\"content\":{\"sides\":[{\"content\":{\"connectorIds\":[\"LConn1\",\"In1\"]},\"type\":\"ConnectorPlacement.EquallySpacedRectSide\",\"uuid\":\"50c89675-cb8a-4964-af62-cb2014507b1d\"},{\"content\":{\"connectorIds\":[\"RConn1\",\"Out1\"],\"side\":\"RIGHT\"},\"type\":\"ConnectorPlacement.EquallySpacedRectSide\",\"uuid\":\"6b3adc78-0be5-4682-9da0-6fd41ffc4e71\"},{\"content\":{\"connectorIds\":[],\"side\":\"TOP\"},\"type\":\"ConnectorPlacement.EquallySpacedRectSide\",\"uuid\":\"5158b46f-a496-48e4-90d6-6c6dcc9e237b\"}]},\"type\":\"ConnectorPlacement.EquallySpacedConnector\",\"uuid\":\"7ff0188e-dc19-44a0-a8cf-bde33949414f\"}],\"packageUris\":[\"http://schema.mathworks.com/mf0/Connector/R2020b\"],\"version\":\"1.0\"}"
  Integrator : Integrator
  PS-Simulink Converter : nesl_utility/PS-Simulink Converter  PhysicalDomain=network_engine_domain  SubClassName=ps_output  LeftPortType=input  RightPortType=output  PseudoPeriodic=off  Frequencies=[]  Unit=inherit  AffineConversion=off
      settings: SourceProductBaseCode=PW,SS
  Product : Product
  VolumeToVoid : Gain  Gain=1/Volume
  Ref1 : PMIOPort  Side=Left
  VolumeRate : PMIOPort  Port=2  Side=Left
  Ref2 : PMIOPort  Port=3  Side=Left
  GasOut : Outport
  wires:
  VolumeToVoid/1 -> Add/2, GasExpansion/1
  Integrator/1 -> VolumeToVoid/1
  GasIn/1 -> Add/1
  Add/1 -> Product/1
  Product/1 -> Integrator/1
  PS-Simulink Converter/1 -> Product/2
  GasExpansion/1 -> GasOut/1
  connections:
  PS-Simulink Converter/LConn1 -- VolumeRate/RConn1
  GasExpansion/LConn1 -- Ref1/RConn1
  GasExpansion/RConn1 -- Ref2/RConn1

== system MSDRPrimaryLoop_LoadFollow/Chemical Processing/PipeLine/PLossFunc ==
  Constant : Constant  Value=pipeLineElevation*9.82
  PS-Simulink Converter : nesl_utility/PS-Simulink Converter  PhysicalDomain=network_engine_domain  SubClassName=ps_output  LeftPortType=input  RightPortType=output  PseudoPeriodic=off  Frequencies=[]  Unit=inherit  AffineConversion=off
      settings: SourceProductBaseCode=PW,SS
  PS-Simulink Converter1 : nesl_utility/PS-Simulink Converter  PhysicalDomain=network_engine_domain  SubClassName=ps_output  LeftPortType=input  RightPortType=output  PseudoPeriodic=off  Frequencies=[]  Unit=inherit  AffineConversion=off
      settings: SourceProductBaseCode=PW,SS
  Pressure & Temperature Sensor (TL) : fl_lib/Thermal Liquid/Sensors/Pressure & Temperature Sensor (TL)
      settings: SourceProductBaseCode=SS  InternalSimscapePortConfiguration="{\"Bottom\":[],\"Left\":[{\"id\":\"A\",\"label\":\"A\",\"type\":\"foundation.thermal_liquid.thermal_liquid\"}],\"Right\":[{\"id\":\"B\",\"label\":\"B\",\"type\":\"foundation.thermal_liquid.thermal_liquid\"},{\"id\":\"P\",\"label\":\"P\",\"type\":\"output\"},{\"id\":\"T\",\"label\":\"T\",\"type\":\"output\"}],\"Top\":[]}"
  Product : Product
  Subtract : Sum  Inputs=+-
  Thermodynamic Properties Sensor (TL) : fl_lib/Thermal Liquid/Sensors/Thermodynamic Properties Sensor (TL)
      settings: SourceProductBaseCode=SS  InternalSimscapePortConfiguration="{\"Bottom\":[],\"Left\":[{\"id\":\"A\",\"label\":\"A\",\"type\":\"foundation.thermal_liquid.thermal_liquid\"}],\"Right\":[{\"id\":\"U\",\"label\":\"u\",\"type\":\"output\"},{\"id\":\"RHO\",\"label\":\"rho\",\"type\":\"output\"},{\"id\":\"CP\",\"label\":\"cp\",\"type\":\"output\"}],\"Top\":[]}"
  Ref1 : PMIOPort  Side=Left
  Ref2 : PMIOPort  Port=2  Side=Right
  PLoss : Outport
  wires:
  PS-Simulink Converter1/1 -> Product/1
  PS-Simulink Converter/1 -> Subtract/1
  Product/1 -> Subtract/2
  Constant/1 -> Product/2
  Subtract/1 -> PLoss/1
  connections:
  Thermodynamic Properties Sensor (TL)/LConn1 -- Pressure & Temperature Sensor (TL)/RConn1 -- Ref2/RConn1
  PS-Simulink Converter/LConn1 -- Pressure & Temperature Sensor (TL)/RConn2
  Thermodynamic Properties Sensor (TL)/RConn2 -- PS-Simulink Converter1/LConn1
  Pressure & Temperature Sensor (TL)/LConn1 -- Ref1/RConn1
